simulink model "PMSM_FOC_demo"  (R2016a)
settings: Solver=ode3  StartTime=0.0  StopTime=0.4  FixedStep=ts  RelTol=1e-3
InitFcn:
  | para_init;
values from neighbouring files (symbols this model uses):
  J = 0.15    [para_init.m]
  MotOpMod = 2    [para_init.m]
  n_max = 6000    [para_init.m]
  nMotOpSpdMod = 1000*2*pi/60    (= 104.71975512)    [para_init.m]
  pp = 6    [para_init.m]
  r_dq = tan(theta_mtpa)    [para_init.m]
  ts_cc = 1/f_cc    (= 0.0001)    [para_init.m]
  U_bat = 200    [para_init.m]
undefined symbols (not defined in the file or in its folder): sigbuilder_block
undefined symbols (not defined in the file): f_cc, i_max, i_min, Kc_id, Kc_iq, Kc_n, Ki_id, Ki_iq, Ki_n, Kp_id, Kp_iq, Kp_n, Lamda_pm, lpa_cc, lpb_cc, Ls_d, Ls_q, rs, Te_max, Te_min, theta0, ts
libraries: simulink x2, simulink_extras x1
(part 2 of 2)

== stateflow chart PMSM_FOC_demo/MCUPWMGen(TI2812)/PulseFilt ==
  (default) -> (junction 3) : /* PWMPulseFilter PhaseA */
  (junction 3) -> (junction 6) [order 1] : [TaIn<PulseLimlo]
  (junction 3) -> (junction 5) [order 2]
  (junction 6) -> (junction 7) : {TaOut=0;}
  (junction 5) -> (junction 8) [order 1] : [TaIn>PulseLimup]
  (junction 5) -> (junction 4) [order 2] : {TaOut=TaIn;}
  (junction 8) -> (junction 9) : {TaOut=nMax;}
  (junction 9) -> (junction 4)
  (junction 7) -> (junction 9)
  (junction 4) -> (junction 30) : /* PWMPulseFilter  PhaseB*/
  (junction 30) -> (junction 33) [order 1] : [TbIn<PulseLimlo]
  (junction 30) -> (junction 32) [order 2]
  (junction 33) -> (junction 34) : {TbOut=0;}
  (junction 32) -> (junction 35) [order 1] : [TbIn>PulseLimup]
  (junction 32) -> (junction 31) [order 2] : {TbOut=TbIn;}
  (junction 35) -> (junction 36) : {TbOut=nMax;}
  (junction 36) -> (junction 31)
  (junction 34) -> (junction 36)
  (junction 31) -> (junction 47) : /* PWMPulseFilter  PhaseC*/
  (junction 47) -> (junction 50) [order 1] : [TcIn<PulseLimlo]
  (junction 47) -> (junction 49) [order 2]
  (junction 50) -> (junction 51) : {TcOut=0;}
  (junction 49) -> (junction 52) [order 1] : [TcIn>PulseLimup]
  (junction 49) -> (junction 48) [order 2] : {TcOut=TcIn;}
  (junction 52) -> (junction 53) : {TcOut=nMax;}
  (junction 53) -> (junction 48)
  (junction 51) -> (junction 53)
  (junction 48) -> (junction 64)
  data: TaIn input; TbIn input; TcIn input; TaOut output; TbOut output; TcOut output; nMax input; PulseLimup input; PulseLimlo input
